simulink model "Weather_testModel"  (R2020a)
settings: Solver=FixedStepDiscrete  StartTime=0.0  StopTime=10.0  FixedStep=1  RelTol=1e-3
undefined symbols (not defined in the file or in its folder): sigbuilder_block
settings Model: Creator=SAMEEKSHA  LastModifiedBy=SAMEEKSHA
settings ConfigComp: CovEnable=on  RecordCoverage=on  CovMetricSettings=dcmwe  CovModelRefEnable=on

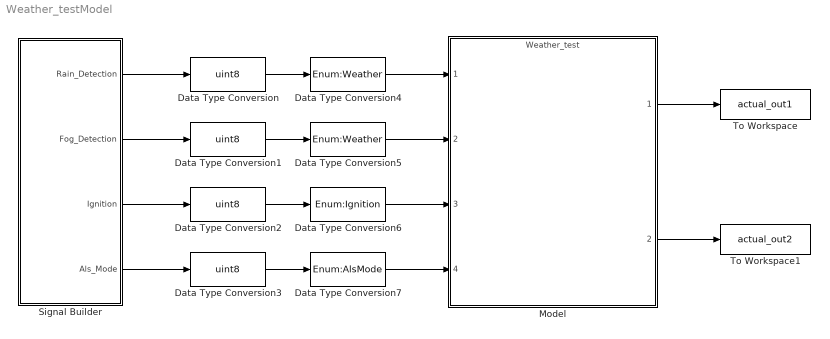
== system Weather_testModel ==
  Data Type Conversion{,1..3} (4 alike) : DataTypeConversion  OutDataTypeStr=uint8  SaturateOnIntegerOverflow=on  LockScale=on
  Data Type Conversion4 : DataTypeConversion  OutDataTypeStr=Enum:Weather  SaturateOnIntegerOverflow=on  LockScale=on
  Data Type Conversion5 : DataTypeConversion  OutDataTypeStr=Enum:Weather  SaturateOnIntegerOverflow=on  LockScale=on
  Data Type Conversion6 : DataTypeConversion  OutDataTypeStr=Enum:Ignition  SaturateOnIntegerOverflow=on  LockScale=on
  Data Type Conversion7 : DataTypeConversion  OutDataTypeStr=Enum:AlsMode  SaturateOnIntegerOverflow=on  LockScale=on
  Model : ModelReference  ModelNameDialog=Weather_test.slx  SimulationMode=Normal  ModelReferenceVersion=1.12
  Signal Builder : Subsystem  Tag=STV Subsys  LoadFcn=sigbuilder_block('load');  StartFcn=sigbuilder_block('start');  StopFcn=sigbuilder_block('stop');  ClipboardFcn=sigbuilder_block('clipboard');  mask(Sigbuilder block){tuvar=[0:10]}
      mask help: Simulink:masks:SigbuilderBlock_MD
      mask init:
      | if ~strcmp(get_param(bdroot(gcbh),'SimulationStatus'),'stopped') tuvar = sigbuilder_block('maskInit'); end
      settings: CopyFcn=sigbuilder_block('copy');  DeleteFcn=sigbuilder_block('delete');  ModelCloseFcn=sigbuilder_block('modelClose');  PreSaveFcn=sigbuilder_block('preSave');  PauseFcn=sigbuilder_block('pause');  ContinueFcn=sigbuilder_block('continue');  NameChangeFcn=sigbuilder_block('namechange');  OpenFcn=sigbuilder_block('open',[437.6 153 550.4 359.25 ]);  CloseFcn=sigbuilder_block('close');
      mask Display: plot(0, 0, 100, 100,[2, 2, 32, 32, 2], [68, 8, 8, 68, 68],[32, 2], [38, 38], [32, 19, 2],[53, 60, 44], [32, 17, 17, 2],[16, 16, 31, 31]);txt = getActiveGroup(gcbh);text(2, 100, txt,'verticalAlignment', 'top');
  To Workspace : ToWorkspace  VariableName=actual_out1  SaveFormat=Timeseries  SampleTime=-1
  To Workspace1 : ToWorkspace  VariableName=actual_out2  SaveFormat=Timeseries  SampleTime=-1
  wires:
  Signal Builder/1(Rain_Detection) -> Data Type Conversion/1
  Signal Builder/2(Fog_Detection) -> Data Type Conversion1/1
  Signal Builder/3(Ignition) -> Data Type Conversion2/1
  Signal Builder/4(Als_Mode) -> Data Type Conversion3/1
  Data Type Conversion/1 -> Data Type Conversion4/1
  Data Type Conversion1/1 -> Data Type Conversion5/1
  Data Type Conversion2/1 -> Data Type Conversion6/1
  Data Type Conversion3/1 -> Data Type Conversion7/1
  Data Type Conversion4/1 -> Model/1
  Data Type Conversion5/1 -> Model/2
  Data Type Conversion6/1 -> Model/3
  Data Type Conversion7/1 -> Model/4
  Model/1 -> To Workspace/1
  Model/2 -> To Workspace1/1

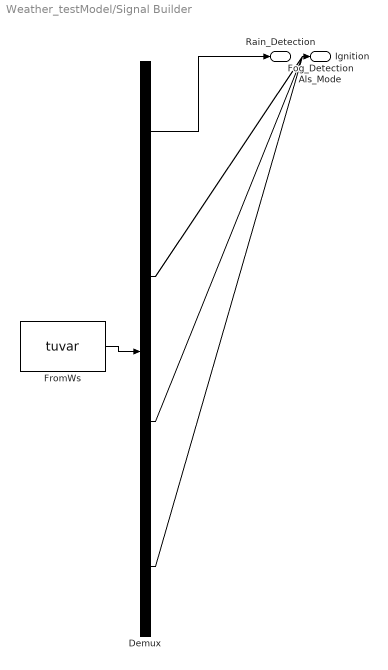
== system Weather_testModel/Signal Builder ==
  Demux : Demux  Tag=STV Demux
      settings: DisplayOption=none
  FromWs : FromWorkspace  Tag=STV FromWs  VariableName=tuvar
      SigBuilderData=|
      | common.afterFinalStr = 'Extrapolate'
      | common.sampleTime = 0
      | dataSet.timeRange = [0 10]
      | dataSet.name = 'Group 1'
      | sbobj.Groups.Name = 'Group 1'
      | sbobj.Groups.Signals(1).Name = 'Rain_Detection'
      | sbobj.Groups.Signals(1).XData = [0 1 2 3 4 5 10]
      | sbobj.Groups.Signals(1).YData = [6 7 6 7 6 7 7]
      | sbobj.Groups.Signals(2).Name = 'Fog_Detection'
      | sbobj.Groups.Signals(2).XData = [0 1 2 3 4 10]
      | sbobj.Groups.Signals(2).YData = [8 8 9 9 8 8]
      | sbobj.Groups.Signals(3).Name = 'Ignition'
      | sbobj.Groups.Signals(3).XData = [0 1 2 3 4 5 10]
      | sbobj.Groups.Signals(3).YData = [0 0 0 0 1 0 0]
      | sbobj.Groups.Signals(4).Name = 'Als_Mode'
      | sbobj.Groups.Signals(4).XData = [0 1 2 3 4 5 10]
      | sbobj.Groups.Signals(4).YData = [0 0 0 0 0 1 1]
  Rain_Detection : Outport  Tag=STV Outport
  Fog_Detection : Outport  Tag=STV Outport  Port=2
  Ignition : Outport  Tag=STV Outport  Port=3
  Als_Mode : Outport  Tag=STV Outport  Port=4
  wires:
  FromWs/1 -> Demux/1
  Demux/1 -> Rain_Detection/1
  Demux/2 -> Fog_Detection/1
  Demux/3 -> Ignition/1
  Demux/4 -> Als_Mode/1
